simulink model "Ejercicio2Difuso2"  (R2024b)
settings: Solver=VariableStepAuto  StartTime=0.0  StopTime=10.0  RelTol=1e-3
settings Model: Creator=user  LastModifiedBy=user

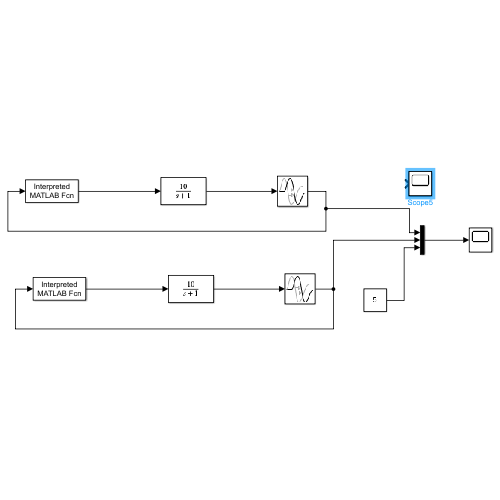
[thumbnail: Simulink's stored preview of the top-level diagram]
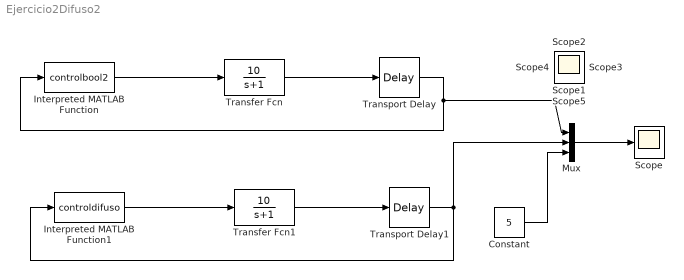
== system Ejercicio2Difuso2 ==
  Constant : Constant  Value=5
  Interpreted MATLAB Function : MATLABFcn  MATLABFcn=controlbool2
  Interpreted MATLAB Function1 : MATLABFcn  MATLABFcn=controldifuso
  Mux : Mux  Inputs=3
  Scope{,1..5} (6 alike) : Scope
  Transfer Fcn : TransferFcn  Numerator=[10]  Denominator=[1 1]
  Transfer Fcn1 : TransferFcn  Numerator=[10]  Denominator=[1 1]
  Transport Delay : TransportDelay  DelayTime=0.5
  Transport Delay1 : TransportDelay  DelayTime=0.5
  wires:
  Interpreted MATLAB Function/1 -> Transfer Fcn/1
  Transfer Fcn/1 -> Transport Delay/1
  Transport Delay/1 -> Interpreted MATLAB Function/1, Mux/1
  Transport Delay1/1 -> Mux/2, Interpreted MATLAB Function1/1
  Transfer Fcn1/1 -> Transport Delay1/1
  Interpreted MATLAB Function1/1 -> Transfer Fcn1/1
  Constant/1 -> Mux/3
  Mux/1 -> Scope/1
